simulink subsystem "ControlReactivo"  (R2023b)
settings: Solver=VariableStepAuto  StartTime=0.0  StopTime=10.0  RelTol=1e-3
settings Model: Creator=Usuario_UMA  LastModifiedBy=Usuario_UMA

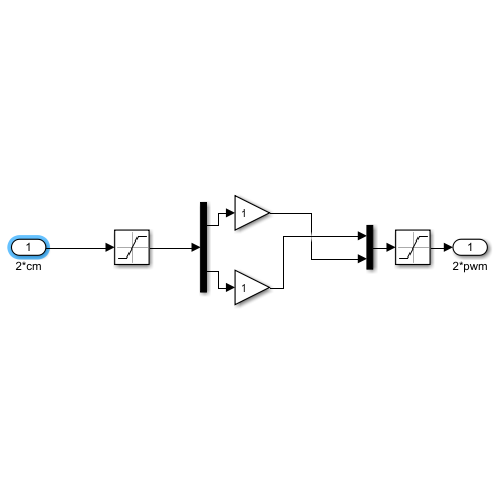
[thumbnail: Simulink's stored preview of the top-level diagram]
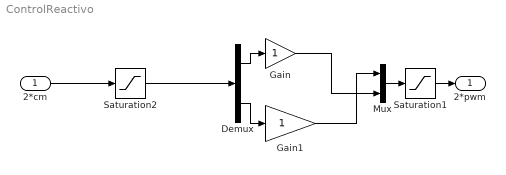
== system ControlReactivo ==
  2*cm : Inport
  Demux : Demux  Outputs=2
  Gain : Gain
  Gain1 : Gain
  Mux : Mux  Inputs=2
  Saturation1 : Saturate  UpperLimit=150  LowerLimit=0  OutDataTypeStr=int16
  Saturation2 : Saturate  UpperLimit=150  LowerLimit=0
  2*pwm : Outport
  wires:
  2*cm/1 -> Saturation2/1
  Saturation1/1 -> 2*pwm/1
  Gain/1 -> Mux/2
  Mux/1 -> Saturation1/1
  Demux/1 -> Gain/1
  Gain1/1 -> Mux/1
  Demux/2 -> Gain1/1
  Saturation2/1 -> Demux/1
